simulink model "ProposedProblem2"  (R2013a)
settings: Solver=ode45  StartTime=0.0  StopTime=604800  RelTol=1e-3
undefined symbols (not defined in the file): des, gcbh
settings Model: Creator=gabig  LastModifiedBy=gabig

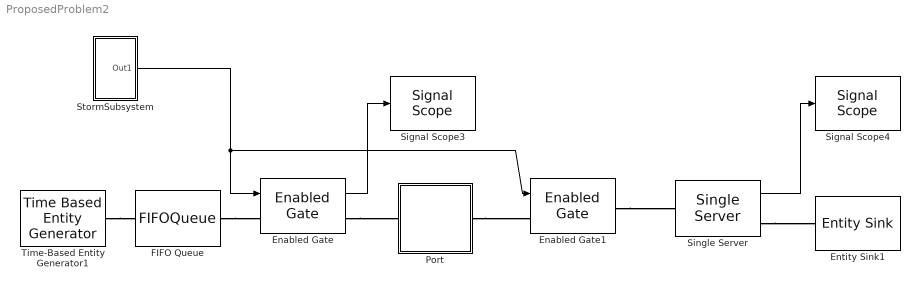
== system ProposedProblem2 ==
  Enabled Gate : EnabledGate  StatNumberDeparted=on
  Enabled Gate1 : EnabledGate
  Entity Sink1 : EntitySink
  FIFO Queue : FIFOQueue
  Port : Subsystem
  Signal Scope3 : SignalScope  LoadFcn=des.scope.CallbackSupport('seLoadFcn',gcbh)  StartFcn=des.scope.CallbackSupport('seStartFcn',gcbh)  StopFcn=des.scope.CallbackSupport('seStopFcn',gcbh)
      settings: CopyFcn=des.scope.CallbackSupport('seCopyFcn',gcbh)  DeleteFcn=des.scope.CallbackSupport('seDeleteFcn',gcbh)  PreSaveFcn=des.scope.CallbackSupport('sePreSaveFcn',gcbh)  NameChangeFcn=des.scope.CallbackSupport('seNameChangeFcn',gcbh)  OpenFcn=des.scope.CallbackSupport('seOpenFcn',gcbh)
  Signal Scope4 : SignalScope  LoadFcn=des.scope.CallbackSupport('seLoadFcn',gcbh)  StartFcn=des.scope.CallbackSupport('seStartFcn',gcbh)  StopFcn=des.scope.CallbackSupport('seStopFcn',gcbh)
      settings: CopyFcn=des.scope.CallbackSupport('seCopyFcn',gcbh)  DeleteFcn=des.scope.CallbackSupport('seDeleteFcn',gcbh)  PreSaveFcn=des.scope.CallbackSupport('sePreSaveFcn',gcbh)  NameChangeFcn=des.scope.CallbackSupport('seNameChangeFcn',gcbh)  OpenFcn=des.scope.CallbackSupport('seOpenFcn',gcbh)
  Single Server : SingleServer  ServiceTime=1800  StatNumberDeparted=on
  StormSubsystem : Subsystem
  Time-Based Entity Generator1 : TimeBasedEntityGenerator  Distribution=Uniform  InitialSeed=12346  Minimum=10800  Maximum=18000
  wires:
  Enabled Gate/1 -> Signal Scope3/1
  StormSubsystem/1(Out1) -> Enabled Gate/1, Enabled Gate1/1
  Single Server/1 -> Signal Scope4/1
  connections:
  Enabled Gate/RConn1 -- Port/LConn1
  Port/RConn1 -- Enabled Gate1/LConn1
  Time-Based Entity Generator1/RConn1 -- FIFO Queue/LConn1
  Single Server/RConn1 -- Entity Sink1/LConn1
  FIFO Queue/RConn1 -- Enabled Gate/LConn1
  Enabled Gate1/RConn1 -- Single Server/LConn1

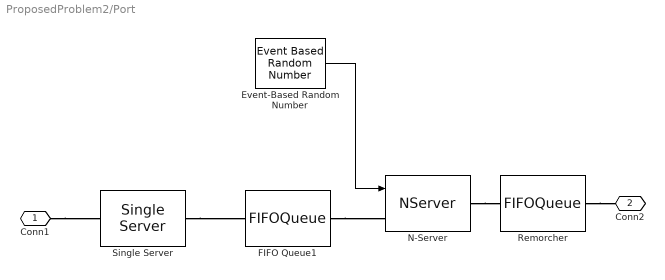
== system ProposedProblem2/Port ==
  Event-Based Random Number : EventBasedRandomNumber  Distribution=Uniform  minUnif=25200  maxUnif=61200
  FIFO Queue1 : FIFOQueue
  N-Server : NServer  NumberOfServers=3  ServiceTimeFrom=Signal port t
  Remorcher : FIFOQueue
  Single Server : SingleServer  ServiceTime=3600
  Conn1 : PMIOPort  Port=1  Side=Left
  Conn2 : PMIOPort  Port=2  Side=Right
  wires:
  Event-Based Random Number/1 -> N-Server/1
  connections:
  Remorcher/RConn1 -- Conn2/RConn1
  Single Server/RConn1 -- FIFO Queue1/LConn1
  Conn1/RConn1 -- Single Server/LConn1
  FIFO Queue1/RConn1 -- N-Server/LConn1
  N-Server/RConn1 -- Remorcher/LConn1

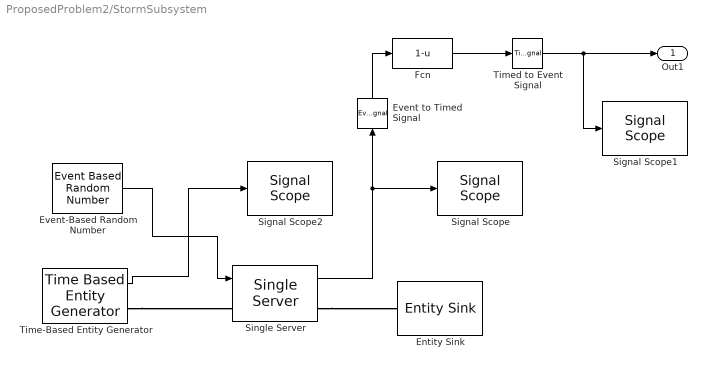
== system ProposedProblem2/StormSubsystem ==
  Entity Sink : EntitySink
  Event to Timed Signal : EventToTimedSignal
  Event-Based Random Number : EventBasedRandomNumber  Distribution=Uniform  minUnif=7200  maxUnif=21600  Seed=12385
  Fcn : Fcn  Expr=1-u
  Signal Scope : SignalScope  LoadFcn=des.scope.CallbackSupport('seLoadFcn',gcbh)  StartFcn=des.scope.CallbackSupport('seStartFcn',gcbh)  StopFcn=des.scope.CallbackSupport('seStopFcn',gcbh)
      settings: CopyFcn=des.scope.CallbackSupport('seCopyFcn',gcbh)  DeleteFcn=des.scope.CallbackSupport('seDeleteFcn',gcbh)  PreSaveFcn=des.scope.CallbackSupport('sePreSaveFcn',gcbh)  NameChangeFcn=des.scope.CallbackSupport('seNameChangeFcn',gcbh)  OpenFcn=des.scope.CallbackSupport('seOpenFcn',gcbh)
  Signal Scope1 : SignalScope  LoadFcn=des.scope.CallbackSupport('seLoadFcn',gcbh)  StartFcn=des.scope.CallbackSupport('seStartFcn',gcbh)  StopFcn=des.scope.CallbackSupport('seStopFcn',gcbh)
      settings: CopyFcn=des.scope.CallbackSupport('seCopyFcn',gcbh)  DeleteFcn=des.scope.CallbackSupport('seDeleteFcn',gcbh)  PreSaveFcn=des.scope.CallbackSupport('sePreSaveFcn',gcbh)  NameChangeFcn=des.scope.CallbackSupport('seNameChangeFcn',gcbh)  OpenFcn=des.scope.CallbackSupport('seOpenFcn',gcbh)
  Signal Scope2 : SignalScope  LoadFcn=des.scope.CallbackSupport('seLoadFcn',gcbh)  StartFcn=des.scope.CallbackSupport('seStartFcn',gcbh)  StopFcn=des.scope.CallbackSupport('seStopFcn',gcbh)
      settings: CopyFcn=des.scope.CallbackSupport('seCopyFcn',gcbh)  DeleteFcn=des.scope.CallbackSupport('seDeleteFcn',gcbh)  PreSaveFcn=des.scope.CallbackSupport('sePreSaveFcn',gcbh)  NameChangeFcn=des.scope.CallbackSupport('seNameChangeFcn',gcbh)  OpenFcn=des.scope.CallbackSupport('seOpenFcn',gcbh)
  Single Server : SingleServer  ServiceTimeFrom=Signal port t  StatNumberInBlock=on
      settings: OutputPortMap=o1
  Time-Based Entity Generator : TimeBasedEntityGenerator  Distribution=Uniform  Minimum=158400  Maximum=187200  StatNumberDeparted=on
  Timed to Event Signal : TimedToEventSignal
  Out1 : Outport
  wires:
  Event to Timed Signal/1 -> Fcn/1
  Time-Based Entity Generator/1 -> Signal Scope2/1
  Fcn/1 -> Timed to Event Signal/1
  Timed to Event Signal/1 -> Signal Scope1/1, Out1/1
  Single Server/1 -> Event to Timed Signal/1, Signal Scope/1
  Event-Based Random Number/1 -> Single Server/1
  connections:
  Single Server/RConn1 -- Entity Sink/LConn1
  Time-Based Entity Generator/RConn1 -- Single Server/LConn1
